simulink model "Concatenate5"  (R2017b)
settings: Solver=FixedStepAuto  StartTime=0.0  StopTime=0  FixedStep=0.1  MaxStep=1  RelTol=1e-3  EnableMultiTasking=on
settings Model: Creator=arnaud  LastModifiedBy=hbourbou
settings DataIOCC: LimitDataPoints=on  SaveFormat=Structure
settings OptimizationCC: LifeSpan=inf
settings DebuggingCC: SolverPrmCheckMsg=warning  SFUnexpectedBacktrackingDiag=warning  SFNoUnconditionalDefaultTransitionDiag=warning  SFExecutionAtInitializationDiag=none
settings HardwareCC: ProdBitPerPointer=32  ProdBitPerSizeT=32  ProdBitPerPtrDiffT=32  ProdLargestAtomicFloat=None  ProdIntDivRoundTo=Undefined  ProdEndianess=Unspecified  ProdWordSize=32  ProdHWDeviceType=32-bit Generic
settings ModelReferenceCC: PropagateSignalLabelsOutOfModel=off
settings CodeAppCC: StateflowObjectComments=on
settings GRTTargetCC: TargetLangStandard=C89/C90 (ANSI)  GeneratePreprocessorConditionals=Disable all
settings ConfigComp: CovMetricSettings=dw  CovHtmlReporting=on  CovSaveCumulativeToWorkspaceVar=on  CovSaveSingleToWorkspaceVar=on  CovExternalEMLEnable=off  CovSFcnEnable=off

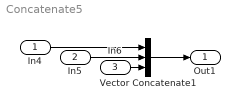
== system Concatenate5 ==
  In4 : Inport  OutDataTypeStr=double
  In5 : Inport  Port=2  OutDataTypeStr=double  PortDimensions=5
  In6 : Inport  Port=3  OutDataTypeStr=double
  Vector Concatenate1 : Concatenate  NumInputs=3
  Out1 : Outport
  wires:
  Vector Concatenate1/1 -> Out1/1
  In4/1 -> Vector Concatenate1/1
  In5/1 -> Vector Concatenate1/2
  In6/1 -> Vector Concatenate1/3
